simulink library "GESHandler"  (R2016b)
settings: Solver=VariableStepAuto  StartTime=0.0  StopTime=10.0  RelTol=1e-3
settings Model: Creator=Nathan  LastModifiedBy=march

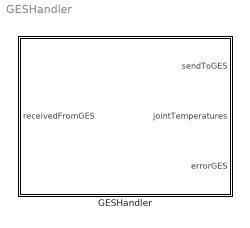
== system GESHandler ==
  GESHandler : Subsystem

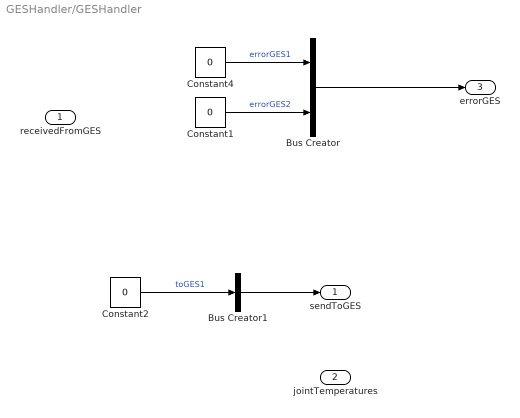
== system GESHandler/GESHandler ==
  receivedFromGES : Inport  OutDataTypeStr=Bus: inGES  BusOutputAsStruct=on
  Bus Creator : BusCreator  Inputs=2
  Bus Creator1 : BusCreator  Inputs=1
  Constant1 : Constant  Value=0
      settings: OpenFcn=|
      | b = get_param(gcb,'value');
      | if (strcmp(b,'72')),
      |   set_param (gcb,'value','0');
      | else
      |   set_param(gcb,'value','72');
      | end;
  Constant2 : Constant  Value=0
      settings: OpenFcn=|
      | b = get_param(gcb,'value');
      | if (strcmp(b,'1')),
      |   set_param (gcb,'value','0');
      | else
      |   set_param(gcb,'value','1');
      | end;
  Constant4 : Constant  Value=0
      settings: OpenFcn=|
      | b = get_param(gcb,'value');
      | if (strcmp(b,'72')),
      |   set_param (gcb,'value','0');
      | else
      |   set_param(gcb,'value','72');
      | end;
  sendToGES : Outport
  jointTemperatures : Outport  Port=2
  errorGES : Outport  Port=3
  wires:
  Bus Creator1/1 -> sendToGES/1
  Constant2/1 -> Bus Creator1/1  "toGES1"
  Bus Creator/1 -> errorGES/1
  Constant4/1 -> Bus Creator/1  "errorGES1"
  Constant1/1 -> Bus Creator/2  "errorGES2"
